simulink library "LibDBC_SCU_ch1"  (R2024b)
settings: Solver=VariableStepAuto  StartTime=0.0  StopTime=10.0  RelTol=1e-3
undefined symbols (not defined in the file): bit_packing, bit_unpacking, IO_Blk_Lib_TTC500, IO_CAN_ConfigMsg, IO_CAN_ReadMsg
libraries: simulink x59, IOBlock_Library_TTC580 x32
(part 1 of 21)
Description:
  | 06-Nov-2024 18:43:00125937
settings Model: Creator=Jacob  LastModifiedBy=Jacob

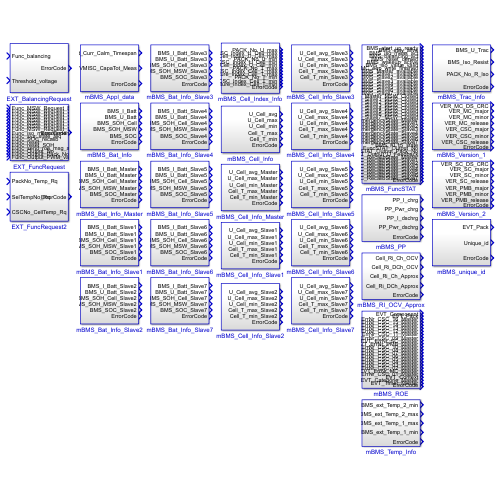
[thumbnail: Simulink's stored preview of the top-level diagram]
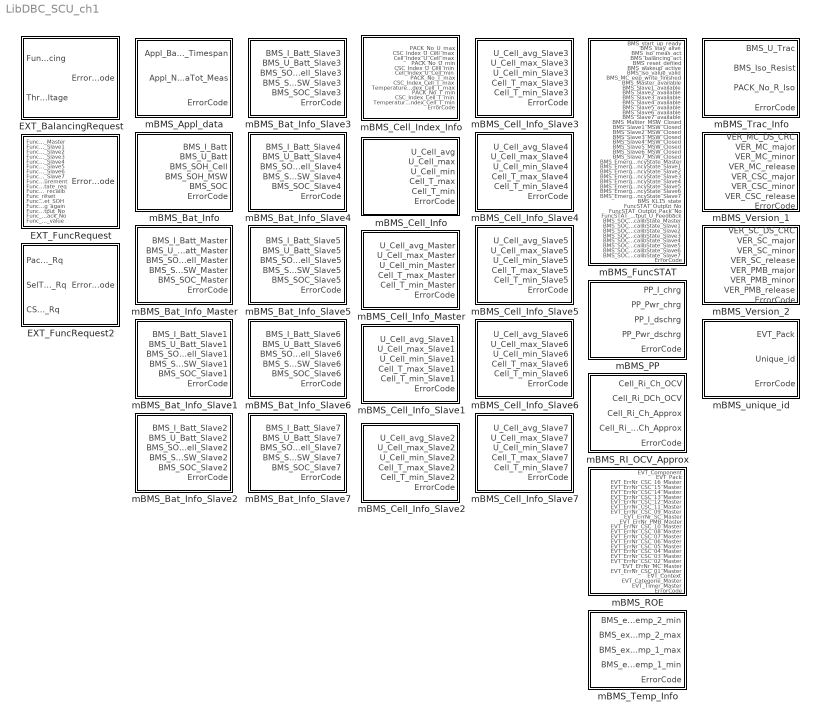
== system LibDBC_SCU_ch1 ==
  EXT_BalancingRequest : Subsystem  Priority=0
  EXT_FuncRequest : Subsystem  Priority=0
  EXT_FuncRequest2 : Subsystem  Priority=0
  mBMS_Appl_data : Subsystem  Priority=0
  mBMS_Bat_Info : Subsystem  Priority=0
  mBMS_Bat_Info_Master : Subsystem  Priority=0
  mBMS_Bat_Info_Slave1 : Subsystem  Priority=0
  mBMS_Bat_Info_Slave2 : Subsystem  Priority=0
  mBMS_Bat_Info_Slave3 : Subsystem  Priority=0
  mBMS_Bat_Info_Slave4 : Subsystem  Priority=0
  mBMS_Bat_Info_Slave5 : Subsystem  Priority=0
  mBMS_Bat_Info_Slave6 : Subsystem  Priority=0
  mBMS_Bat_Info_Slave7 : Subsystem  Priority=0
  mBMS_Cell_Index_Info : Subsystem  Priority=0
  mBMS_Cell_Info : Subsystem  Priority=0
  mBMS_Cell_Info_Master : Subsystem  Priority=0
  mBMS_Cell_Info_Slave1 : Subsystem  Priority=0
  mBMS_Cell_Info_Slave2 : Subsystem  Priority=0
  mBMS_Cell_Info_Slave3 : Subsystem  Priority=0
  mBMS_Cell_Info_Slave4 : Subsystem  Priority=0
  mBMS_Cell_Info_Slave5 : Subsystem  Priority=0
  mBMS_Cell_Info_Slave6 : Subsystem  Priority=0
  mBMS_Cell_Info_Slave7 : Subsystem  Priority=0
  mBMS_FuncSTAT : Subsystem  Priority=0
  mBMS_PP : Subsystem  Priority=0
  mBMS_RI_OCV_Approx : Subsystem  Priority=0
  mBMS_ROE : Subsystem  Priority=0
  mBMS_Temp_Info : Subsystem  Priority=0
  mBMS_Trac_Info : Subsystem  Priority=0
  mBMS_Version_1 : Subsystem  Priority=0
  mBMS_Version_2 : Subsystem  Priority=0
  mBMS_unique_id : Subsystem  Priority=0

== system LibDBC_SCU_ch1/EXT_BalancingRequest ==
  note: Don't change the Names of the Blocks
  Func_balancing : Inport
  Threshold_voltage : Inport  Port=2
  IO_CAN_ConfigMsg : Subsystem  mask(IO_CAN_ConfigMsg_Code){SampleTime=-1, ttlib=IO_Blk_Lib_TTC500, ttDescription=IO_CAN_ConfigMsg, tt_iolib_version=0.19, channel=IO_CAN_CHANNEL_1, mode=IO_CAN_MSG_WRITE, id_format=IO_CAN_STD_FRAME, id=0x7FE, ac_mask=0x7FF}
      mask help: Configures a message object for the given CAN channel.
      mask init:
      | %
      mask Help: web(which('IO_CAN.h'))
      mask TypeOptions channel: IO_CAN_CHANNEL_0  | IO_CAN_CHANNEL_1 | IO_CAN_CHANNEL_2 | IO_CAN_CHANNEL_3 | IO_CAN_CHANNEL_4 | IO_CAN_CHANNEL_5 | IO_CAN_CHANNEL_6
      mask Callback channel: %
      mask TypeOptions mode: IO_CAN_MSG_READ | IO_CAN_MSG_WRITE
      mask Callback mode: %
      mask TypeOptions id_format: IO_CAN_STD_FRAME | IO_CAN_EXT_FRAME
      mask Callback id_format: %
      mask Callback id: %
      mask Callback ac_mask: %
  IO_CAN_WriteMsg : IOBlock_Library_TTC580/CAN  Blocks TTC580 IOlib/WriteMsg_CAN/IO_CAN_WriteMsg  SampleTime=-1  ttlib=IO_Blk_Lib_TTC500  ttDescription=IO_CAN_WriteMsg  tt_iolib_version=0.19
      settings: SourceProductName=I/O Blocklibrary for TTC580
  OR_TX : simulink/Logic and Bit Operations/Bitwise Operator  logicop=OR  UseBitMask=off  NumInputPorts=2  BitMask=bin2dec('11011001')  BitMaskRealWorld=Stored Integer
  Terminator5 : Terminator
  bit_packing1 : Subsystem  LoadFcn=|  mask(bit_packing_Code){SampleTime=-1, ttlib=IO_Blk_Lib_TTC500, ttDescription=bit_packing, tt_iolib_version=0.26, Endianness=little, Format=unsigned, Inversion=off, Startbit=0, Width_bits=8, Factor=1, Offset=0}
      | try
      | %
      | %Upgrade Information - standard BEGIN
      | new_color = 'blue';
      | new_ver = '0.26';
      | act_ver = get_param(gcb,'tt_iolib_version');
      | if not(strcmp(act_ver,new_ver))
      |     disp(['Upgrade block: ',gcb,char(10),'       Version: ',act_ver,' to ',new_ver]);
      |     %switch - case for specific upgrade information e.g. additional parameter required 
      |     %Change appearance and version information
      |     set_param(gcb,'ForegroundColor',new_color);
      |     set_param(gcb,'tt_iolib_version',new_ver);
      | end
      | %Upgrade Information - standard END
      | catch
      | %Standard catch section BEGIN
      | errordlg('An error occurred in a callback of the TTC580-BlockLib. Please open the Diagnostic Viewer for further details');
      | disp(' ');
      | disp('------------------------------------------------------------');
      | disp('An error occurred in a callback of the TTC580-BlockLib.');
      | disp(['Please check the parameters in the mask of ',gcb]);
      | disp('If you do not encounter any violations, then please '); 
      | disp('copy the following lines and report this to support@ttcontrol.com ');
      | disp('<< begin of error message dump >>');
      | disp(['Version of TTC580-BlockLib: ', get_param(gcb,'tt_iolib_version')]);
      | disp(get_param(gcb,'ttDescription'));
      | disp(gcb);
      | x=lasterror;disp(x.message);
      | disp(get_param(gcb,'MaskValues'));
      | disp(version);
      | disp(computer);
      | disp('<< end of error message dump >>');
      | disp('------------------------------------------------------------');
      | disp(' ');
      | %Standard catch section END
      | end
      mask help:
      | Block to prepare CAN-transmition at specified position within 64bit field.
      | For "Factor" and "Offset" the definition of Vector's CANdb applies:
      | [Physical value] = ( [Raw value] * [Factor] ) + [Offset]
      | with Raw value of a signal being the value as it is transmitted in the CAN-network.
      | Verification capabilities are supported.
      mask init:
      | try
      | %%CT>
      | TAG_loc = get_param(gcb,'Tag');
      | if ~isempty(TAG_loc),[~,y]=regexp(TAG_loc,'(^[a-zA-Z0-9_]*)');
      |     if isempty(y) || y~=builtin('length',(TAG_loc)) %don't use length() alone!
      |         error(['The Tag: ',TAG_loc,' needs to start with a letter and may only contain the characters 0-9,a-Z,_ .']);
      | end,end
      | x=find_system(gcbh,'FollowLinks','on','LookUnderMasks','on','BlockType','S-Function');
      | for i=1:builtin('length',(x)) %don't use length() alone!
      |     set_param(x(i),'Tag',TAG_loc);
      | end
      | %<CT%
      | 
      | catch
      | %Standard catch section BEGIN
      | errordlg('An error occurred in a callback of the TTC580-BlockLib. Please open the Diagnostic Viewer for further details');
      | disp(' ');
      | disp('------------------------------------------------------------');
      | disp('An error occurred in a callback of the TTC580-BlockLib.');
      | disp(['Please check the parameters in the mask of ',gcb]);
      | disp('If you do not encounter any violations, then please '); 
      | disp('copy the following lines and report this to support@ttcontrol.com ');
      | disp('<< begin of error message dump >>');
      | disp(['Version of TTC580-BlockLib: ', get_param(gcb,'tt_iolib_version')]);
      | disp(get_param(gcb,'ttDescription'));
      | disp(gcb);
      | x=lasterror;disp(x.message);
      | disp(get_param(gcb,'MaskValues'));
      | disp(version);
      | disp(computer);
      | disp('<< end of error message dump >>');
      | disp('------------------------------------------------------------');
      | disp(' ');
      | %Standard catch section END
      | end
      mask Help: web([which('usermanual.html'),'#',lower(get_param(gcb,'ttDescription'))])
      mask TypeOptions Endianness: big | little
      mask Callback Endianness: %
      mask TypeOptions Format: unsigned | signed | real32
      mask Callback Format: %
      mask Callback Inversion: %
      mask Callback Startbit: %
      mask Callback Width_bits: %
      mask Callback Factor: %
      mask Callback Offset: %
  bit_packing2 : Subsystem  LoadFcn=|  mask(bit_packing_Code){SampleTime=-1, ttlib=IO_Blk_Lib_TTC500, ttDescription=bit_packing, tt_iolib_version=0.26, Endianness=little, Format=unsigned, Inversion=off, Startbit=8, Width_bits=16, Factor=1, Offset=0}
      | try
      | %
      | %Upgrade Information - standard BEGIN
      | new_color = 'blue';
      | new_ver = '0.26';
      | act_ver = get_param(gcb,'tt_iolib_version');
      | if not(strcmp(act_ver,new_ver))
      |     disp(['Upgrade block: ',gcb,char(10),'       Version: ',act_ver,' to ',new_ver]);
      |     %switch - case for specific upgrade information e.g. additional parameter required 
      |     %Change appearance and version information
      |     set_param(gcb,'ForegroundColor',new_color);
      |     set_param(gcb,'tt_iolib_version',new_ver);
      | end
      | %Upgrade Information - standard END
      | catch
      | %Standard catch section BEGIN
      | errordlg('An error occurred in a callback of the TTC580-BlockLib. Please open the Diagnostic Viewer for further details');
      | disp(' ');
      | disp('------------------------------------------------------------');
      | disp('An error occurred in a callback of the TTC580-BlockLib.');
      | disp(['Please check the parameters in the mask of ',gcb]);
      | disp('If you do not encounter any violations, then please '); 
      | disp('copy the following lines and report this to support@ttcontrol.com ');
      | disp('<< begin of error message dump >>');
      | disp(['Version of TTC580-BlockLib: ', get_param(gcb,'tt_iolib_version')]);
      | disp(get_param(gcb,'ttDescription'));
      | disp(gcb);
      | x=lasterror;disp(x.message);
      | disp(get_param(gcb,'MaskValues'));
      | disp(version);
      | disp(computer);
      | disp('<< end of error message dump >>');
      | disp('------------------------------------------------------------');
      | disp(' ');
      | %Standard catch section END
      | end
      mask help:
      | Block to prepare CAN-transmition at specified position within 64bit field.
      | For "Factor" and "Offset" the definition of Vector's CANdb applies:
      | [Physical value] = ( [Raw value] * [Factor] ) + [Offset]
      | with Raw value of a signal being the value as it is transmitted in the CAN-network.
      | Verification capabilities are supported.
      mask init: same as LibDBC_SCU_ch1/EXT_BalancingRequest/bit_packing1
      mask Help: web([which('usermanual.html'),'#',lower(get_param(gcb,'ttDescription'))])
      mask TypeOptions Endianness: big | little
      mask Callback Endianness: %
      mask TypeOptions Format: unsigned | signed | real32
      mask Callback Format: %
      mask Callback Inversion: %
      mask Callback Startbit: %
      mask Callback Width_bits: %
      mask Callback Factor: %
      mask Callback Offset: %
  id_TX : Constant  Value=hex2dec('7FE')  OutDataTypeStr=uint32
  id_format_TX : Constant  Value=0  OutDataTypeStr=Inherit: Inherit via back propagation
  length_TX : Constant  Value=8  OutDataTypeStr=Inherit: Inherit via back propagation
  ErrorCode : Outport  VectorParamsAs1DForOutWhenUnconnected=off
  wires:
  id_TX/1 -> IO_CAN_WriteMsg/5
  id_format_TX/1 -> IO_CAN_WriteMsg/4
  length_TX/1 -> IO_CAN_WriteMsg/3
  IO_CAN_ConfigMsg/2(handle) -> IO_CAN_WriteMsg/1
  IO_CAN_ConfigMsg/1(ErrorCode) -> Terminator5/1
  IO_CAN_WriteMsg/1 -> ErrorCode/1
  Func_balancing/1 -> bit_packing1/1(Data_in)
  bit_packing1/1(Data_out) -> OR_TX/1
  Threshold_voltage/1 -> bit_packing2/1(Data_in)
  bit_packing2/1(Data_out) -> OR_TX/2
  OR_TX/1 -> IO_CAN_WriteMsg/2
